simulink model "atrias_nmm_hardware"  (R2014b)
settings: Solver=ode4  StartTime=0.0  StopTime=inf  FixedStep=sample_time  RelTol=1e-3
undefined symbols (not defined in the file): A_lpf_dtau, B1_lpf_dtau, B2_lpf_dtau, boom_mount_angle, boom_pelvis_offset_angle, c, c_jointstop, contactThr, control_start_time, D12_T, d_y_boom_com_offset, d_y_boom_hip_offset, eref, fcut_contact, FmaxBFSH, FmaxGLU, FmaxHAM, FmaxHFL, FmaxRF, FmaxVAS, g, h_boom, HIP_MTR_MAX_CONT_TORQUE, initial_com_height, initial_dx, K, k_sea, kd_lateral, kd_phi12, kd_phi23, kp_lateral, kp_phi12, kp_phi23, l_boom_projected, L_distribution_switch, L_force_ctrl_switch, L_hip_trq_desired, L_knee_trq_desired, L_sea_input_switch, l_seg, L_stim_gain, L_stim_switch, l_yaw_center_to_pelvis, lambdaHip, lambdaKnee, lateral_offset, lateral_target_angle_left, lateral_target_angle_right, lateral_transition_force, loptBFSH, loptGLU, loptHAM, loptHFL, loptRF, loptVAS, Lphi12_des, Lphi23_des, lslackBFSH, lslackGLU, lslackHAM ... (+69)
libraries: simulink_extras x15, simulink x5, slrtlib x3
(part 1 of 9)
settings Model: BufferReuse=off  Creator=wmartin  LastModifiedBy=ryan
settings SolverCC: EnableConcurrentExecution=on
settings DataIOCC: MaxDataPoints=1000000000  SaveFormat=StructureWithTime
settings OptimizationCC: BlockReduction=off  OptimizeBlockIOStorage=off  BufferReuse=off  GlobalBufferReuse=off  ExpressionFolding=off  ExpressionDepthLimit=2147483647  LocalBlockOutputs=off  SimCompilerOptimization=On
settings DebuggingCC: UnderspecifiedInitializationDetection=Classic  MergeDetectMultiDrivingBlocksExec=none  StateNameClashWarn=warning
settings HardwareCC: ProdIntDivRoundTo=Zero  ProdEndianess=LittleEndian  ProdLongLongMode=on  ProdHWDeviceType=Generic->32-bit x86 compatible
settings ModelReferenceCC: UpdateModelReferenceTargets=IfOutOfDate  EnableParallelModelReferenceBuilds=on
settings RTWCC: SystemTargetFile=slrt.tlc  TemplateMakefile=slrt_default_tmf  Description=Simulink Real-Time  RTWVerbose=off  ProcessScript=slrt_make_rtw_hook  RTWCompilerOptimization=On
settings CodeAppCC: MaxIdLength=256
settings SimulinkRealTimeCC: GeneratePreprocessorConditionals=Disable all  EnableShiftOperators=on  RL32LogBufSizeModifier=100000000

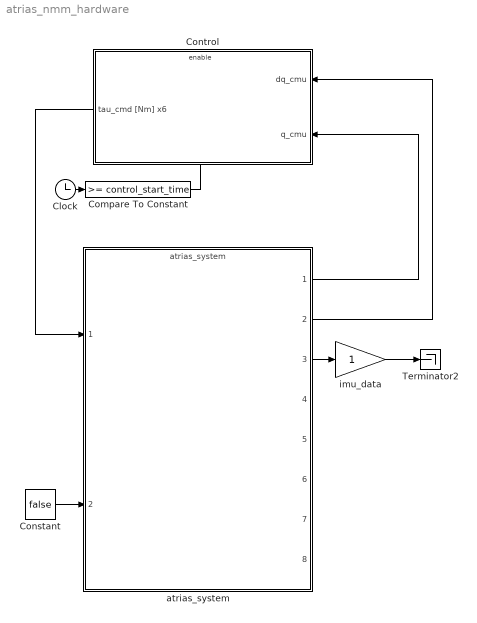
== system atrias_nmm_hardware ==
  Clock : Clock
  Compare To Constant : simulink/Logic and Bit Operations/Compare To Constant  relop=>=  const=control_start_time  OutDataTypeStr=boolean
  Constant : Constant  Value=false
  Control : Subsystem
  Terminator2 : Terminator
  atrias_system : ModelReference  ModelNameDialog=atrias_system  SimulationMode=Normal  ModelReferenceVersion=1.2603  CopyOfModelName=atrias_system  DefaultDataLogging=on
  imu_data : Gain
  wires:
  Clock/1 -> Compare To Constant/1
  Compare To Constant/1 -> Control/Enable
  atrias_system/1 -> Control/2(q_cmu)
  atrias_system/2 -> Control/1(dq_cmu)
  Constant/1 -> atrias_system/2
  Control/1(tau_cmd [Nm] x6) -> atrias_system/1
  imu_data/1 -> Terminator2/1
  atrias_system/3 -> imu_data/1

== system atrias_nmm_hardware/Control ==
  note: (For plotting)
  dq_cmu : Inport
  q_cmu : Inport  Port=2
  Enable : EnablePort  StatesWhenEnabling=reset
  Actuator Control : ModelReference  ModelNameDialog=actuator_control  SimulationMode=Normal  ModelReferenceVersion=1.66  CopyOfModelName=actuator_control  DefaultDataLogging=on
  Behavior Control : Subsystem
  Demux : Demux
  Selector8 : Selector  InputPortWidth=6  Indices=[1 2 4 5]
  tau_cmd [Nm] x6 : Outport  InitialOutput=[0 0 0 0 0 0]
  tag scope: Lshin_cmd_trq=global, Lthigh_cmd_trq=global, Rshin_cmd_trq=global, Rthigh_cmd_trq=global
  wires:
  q_cmu/1 -> Actuator Control/4, Behavior Control/2(q_cmu)
  dq_cmu/1 -> Actuator Control/5, Behavior Control/1(dq_cmu)
  Behavior Control/1(Motor Torque Command [Nm] x6) -> Actuator Control/1
  Actuator Control/1 -> tau_cmd [Nm] x6/1, Selector8/1
  Behavior Control/2(SEA Torque Velocity Command [Nm] x4) -> Actuator Control/2
  Behavior Control/3(Force / Position Control [1/0] x4) -> Actuator Control/3
  Selector8/1 -> Demux/1
  Demux/1 -> [Rshin_cmd_trq]
  Demux/2 -> [Rthigh_cmd_trq]
  Demux/3 -> [Lshin_cmd_trq]
  Demux/4 -> [Lthigh_cmd_trq]
